simulink model "signalAcquisitionR2023b"  (R2023b)
settings: Solver=FixedStepAuto  StartTime=0.0  StopTime=inf  FixedStep=0.01  RelTol=1e-3
model workspace (MAT data in the model file):
  freq = 0.87
settings Model: Creator=marko  LastModifiedBy=marko
settings DebuggingCC: UnconnectedInputMsg=warning  UnconnectedOutputMsg=warning  UnconnectedLineMsg=warning
settings ModelReferenceCC: EnableRefExpFcnMdlSchedulingChecks=on
settings RTWCC: DLArmComputeVersion=19.05
settings ConfigComp: CovBoundaryAbsTol=1.0e-5

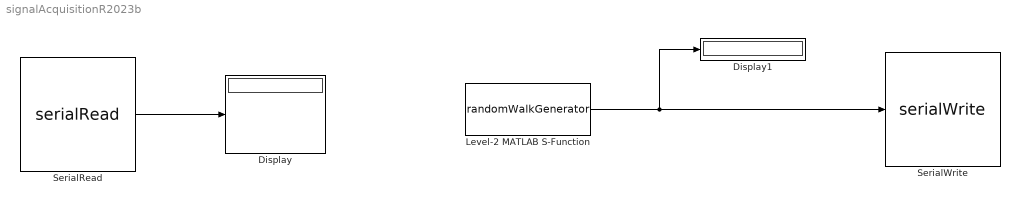
== system signalAcquisitionR2023b ==
  Display : Display
  Display1 : Display
  Level-2 MATLAB S-Function : M-S-Function  FunctionName=randomWalkGenerator
  SerialRead : M-S-Function  FunctionName=serialRead  Parameters='COM4'
  SerialWrite : M-S-Function  FunctionName=serialWrite  Parameters='COM4'
  wires:
  SerialRead/1 -> Display/1
  Level-2 MATLAB S-Function/1 -> Display1/1, SerialWrite/1
